simulink model "Lessons_Scheduled_Completed_v2"  (R2023a)
settings: Solver=VariableStepAuto  StartTime=0.0  StopTime=28  RelTol=1e-3
settings Model: Creator=paulin.kantue  LastModifiedBy=paulin.kantue

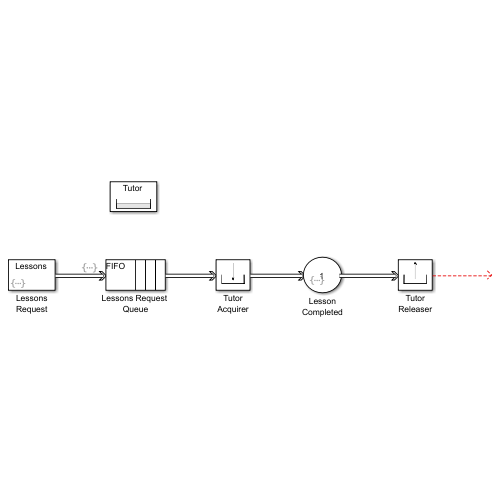
[thumbnail: Simulink's stored preview of the top-level diagram]
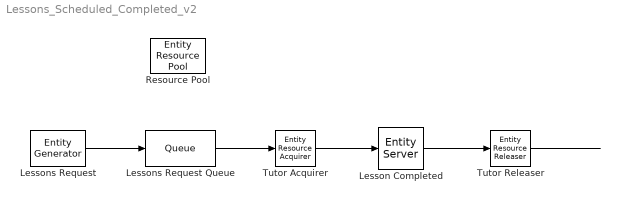
== system Lessons_Scheduled_Completed_v2 ==
  Lesson Completed : EntityServer  InputPortMessageModes=m  OutputPortMessageModes=m  Capacity=1  ServiceCompleteAction=entity.Status = 2; % completed
  Lessons Request : EntityGenerator  OutputPortMessageModes=m  GenerateAction=entity.Status = 0; % requested  AttributeName=Status  AttributeInitialValue=0  EntityType=Structured  EntityTypeName=Lessons
  Lessons Request Queue : Queue  InputPortMessageModes=m  OutputPortMessageModes=m  Capacity=inf  EntryAction=entity.Status = 1; % scheduled
  Resource Pool : EntityResourcePool  ResourceName=Tutor
  Tutor Acquirer : EntityResourceAcquirer  InputPortMessageModes=m  OutputPortMessageModes=m  ResourceName=Tutor
      settings: OutputPortMap=o3
  Tutor Releaser : EntityResourceReleaser  InputPortMessageModes=m  OutputPortMessageModes=m  ResourceToRelease=Selected  ResourceName=Tutor
  wires:
  Lessons Request/1 -> Lessons Request Queue/1
  Lessons Request Queue/1 -> Tutor Acquirer/1
  Tutor Acquirer/1 -> Lesson Completed/1
  Lesson Completed/1 -> Tutor Releaser/1
  Tutor Releaser/1 -> ?
